simulink library "aerolibgravity2"  (R2020a)
settings: Solver=ode45  StartTime=0.0  StopTime=10.0  RelTol=1e-3
PostLoadFcn:
  | load_system('aerolibv1')
  | setsysloc('aerolibv1')
undefined symbols (not defined in the file or in its folder): aeroassertmsg, C, geoidgrid, ghCurrent, GM, latbp, lonbp, minYearCurrent, Newton, nMax10, nMax13, nMaxBetween, nMaxCurrent, R, Raphson, S, svCurrent, tabNMax10, tabNMax13, tabNMaxBetween
libraries: simulink x17, aerolibgravitysys x4
(part 1 of 4)
Description:
  | Aerospace Blockset Library: Gravity
settings Model: FPTRunName=Active  ExtModeAutoUpdateStatusClock=off  Creator=The MathWorks, Inc.  LastModifiedBy=The MathWorks, Inc.
settings DataIOCC: LimitDataPoints=on  SaveFormat=Array  SignalLoggingSaveFormat=ModelDataLogs  ReturnWorkspaceOutputs=off
settings OptimizationCC: BlockReduction=off  BooleanDataType=off  ExpressionDepthLimit=2147483647  EfficientMapNaN2IntZero=off  LifeSpan=inf
settings DebuggingCC: SaveWithParameterizedLinksMsg=none  UnderspecifiedInitializationDetection=Classic  MergeDetectMultiDrivingBlocksExec=none  SignalResolutionControl=TryResolveAllWithWarning  FcnCallInpInsideContextMsg=warning  AllowSymbolicDim=off  StateNameClashWarn=warning  SFUnexpectedBacktrackingDiag=warning  SFNoUnconditionalDefaultTransitionDiag=warning  SFExecutionAtInitializationDiag=none  ArithmeticOperatorsInVariantConditions=warning
settings HardwareCC: ProdBitPerPointer=32  ProdLargestAtomicFloat=None  ProdIntDivRoundTo=Undefined  ProdEndianess=Unspecified  ProdWordSize=32  ProdHWDeviceType=Specified  TargetUnknown=on
settings ModelReferenceCC: PropagateSignalLabelsOutOfModel=off
settings SFSimCC: SimUseLocalCustomCode=off  CustomCodeUndefinedFunction=UseInterfaceOnly
settings RTWCC: RTWUseLocalCustomCode=off
settings CodeAppCC: StateflowObjectComments=on
settings GRTTargetCC: TargetLangStandard=C89/C90 (ANSI)  CombineOutputUpdateFcns=off  GRTInterface=on
settings ConfigComp: CovMetricSettings=dw  CovHtmlReporting=on  CovSaveCumulativeToWorkspaceVar=on  CovSaveSingleToWorkspaceVar=on  CovExternalEMLEnable=off

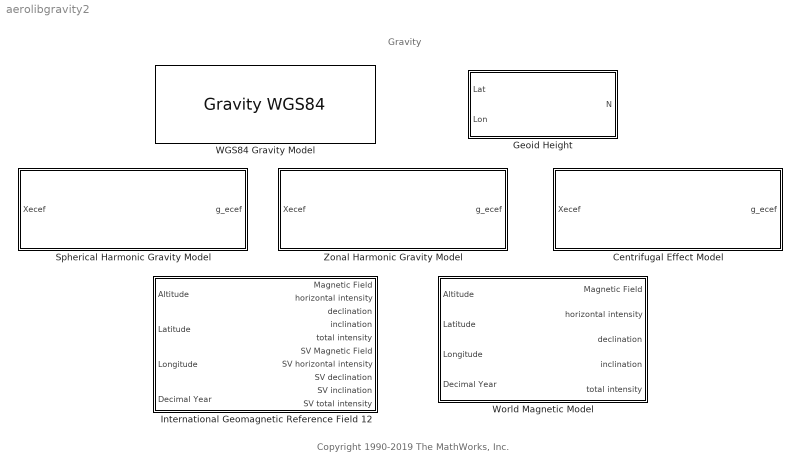
== system aerolibgravity2 ==
  note: Gravity
  note: Copyright 1990-2019 The MathWorks, Inc.
  Centrifugal Effect Model : Subsystem  BlockKeywords=__PRM__SERIALIZED__DATA__:centrifugal force,centrifugal acceleration,Mars,Moon,planet,Mercury,Venus,Jupiter,Saturn,Neptune,Uranus,gravity,rotation,Earth rotation,planetary rotation,non-inertial,noninertial,non inertial  mask(Centrifugal Effect Model){ptype=Earth, omega=7.2921150e-05, rate_loc=off}
      mask prompts: ptype "aeroblks:aeroblkgravity:blockCentrifugalEffectModelParamPlanetmodel"; omega "aeroblks:aeroblkgravity:blockCentrifugalEffectModelParamPlanetaryrotationalrateradsec"; rate_loc "aeroblks:aeroblkgravity:blockCentrifugalEffectModelParamInputplanetaryrotationalrate"
      mask help: aeroblks:aeroblkgravity:blockCentrifugalEffectModelDesc
      mask init:
      | [ports]=aeroicon('aeroblkcentrifugal','icon');
      mask Help: eval('asbhelp');
      mask TypeOptions ptype: aeroblks:aeroblkgravity:blockCentrifugalEffectModelParamComboMercury | aeroblks:aeroblkgravity:blockCentrifugalEffectModelParamComboVenus | aeroblks:aeroblkgravity:blockCentrifugalEffectModelParamComboEarth | aeroblks:aeroblkgravity:blockCentrifugalEffectModelParamComboMoon | aeroblks:aeroblkgravity:blockCentrifugalEffectModelParamComboMars | aeroblks:aeroblkgravity:blockCentrifugalEffectModelParamComboJupiter | aeroblks:aeroblkgravity:blockCentrifugalEffectModelParamComboSaturn | aeroblks:aeroblkgravity:blockCentrifugalEffectModelParamComboUranus | aeroblks:aeroblkgravity:blockCentrifugalEffectModelParamComboNeptune | aeroblks:aeroblkgravity:blockCentrifugalEffectModelParamComboCustom
      mask Callback ptype: aeroicon('aeroblkcentrifugal');
      mask Callback rate_loc: aeroicon('aeroblkcentrifugal');
      mask DialogControl ptype Prompt: Planet model:
      mask DialogControl omega Prompt: Planetary rotational rate [rad/sec]:
      mask DialogControl rate_loc Prompt: Input planetary rotational rate
      mask Display:
      | port_label(ports(1).type,ports(1).port,ports(1).txt,'texmode','on');
      | port_label(ports(2).type,ports(2).port,ports(2).txt,'texmode','on');
      | port_label(ports(3).type,ports(3).port,ports(3).txt,'texmode','on');
  Geoid Height : Subsystem  BlockKeywords=__PRM__SERIALIZED__DATA__:geoidheight,EGM96,EGM2008,geopotential model,WGS84 ellipsoid  mask(Geoid Height){units=Metric (MKS), gtype=EGM96, datafile='geoidegm96grid', dtype=double, action=Warning}
      mask prompts: units "aeroblks:aeroblkgravity:blockGeoidHeightParamUnits"; gtype "aeroblks:aeroblkgravity:blockGeoidHeightParamGeopotentialmodel"; datafile "aeroblks:aeroblkgravity:blockGeoidHeightParamGeopotentialmatfile"; dtype "aeroblks:aeroblkgravity:blockGeoidHeightParamDatatype"; action "aeroblks:aeroblkgravity:blockGeoidHeightParamActionforoutofrangeinput"
      mask help: aeroblks:aeroblkgravity:blockGeoidHeightDesc
      mask init:
      | [ports, latbp, lonbp, geoidgrid, errMode, errData, errSize] = aeroicon('aeroblkgeoidheight','icon');
      | blk = gcb;
      | switch errMode
      |     case 0
      |         % do nothing
      |     case 1
      |         error(message('aeroblks:aeroblkgeoidheight:noDataFile',...
      |                     datafile, blk));
      |     case 2
      |         error(message('aeroblks:aeroblkgeoidheight:noLatBP', ...
      |                     datafile, blk))
      |     case 3
      |         error(message('aeroblks:aeroblkgeoidheight:noLonBP', ...
      |                     datafile, blk))
      |     case 4
      |         error(message('aeroblks:aeroblkgeoidheight:noGrid', ...
      |                     datafile, blk))
      | end
      | switch errData
      |     case 0
      |         % do nothing
      |     case 1
      |         error(message('aeroblks:aeroblkgeoidheight:dataTypeLatLonGrid'));
      | end
      | switch errSize
      |     case 0
      |         % do nothing
      |     case 1
      |         error(message('aeroblks:aeroblkgeoidheight:sizeLatLon'));
      |     case 2
      |         error(message('aeroblks:aeroblkgeoidheight:sizeGrid'))
      |     case 3
      |         error(message('aeroblks:aeroblkgeoidheight:sizeLatLonGrid'))
      | end
      settings: AttributesFormatString=EGM2008 Geoid Data Unavailable
      mask Help: eval('asbhelp');
      mask TypeOptions units: aeroblks:aeroblkgravity:blockGeoidHeightParamComboMetricMKS | aeroblks:aeroblkgravity:blockGeoidHeightParamComboEnglish
      mask TypeOptions gtype: aeroblks:aeroblkgravity:blockGeoidHeightParamComboEGM96 | aeroblks:aeroblkgravity:blockGeoidHeightParamComboEGM2008 | aeroblks:aeroblkgravity:blockGeoidHeightParamComboCustom
      mask Callback gtype: aeroicon('aeroblkgeoidheight');
      mask TypeOptions dtype: aeroblks:aeroblkgravity:blockGeoidHeightParamCombodouble | aeroblks:aeroblkgravity:blockGeoidHeightParamCombosingle
      mask TypeOptions action: aeroblks:aeroblkgravity:blockGeoidHeightParamComboNone | aeroblks:aeroblkgravity:blockGeoidHeightParamComboWarning | aeroblks:aeroblkgravity:blockGeoidHeightParamComboError
      mask DialogControl units Prompt: Units:
      mask DialogControl gtype Prompt: Geopotential model:
      mask DialogControl getdata Prompt: aeroblks:aeroblkgeoidheight:getDataButton
      mask DialogControl getdata Callback: aeroDataPackage
      mask DialogControl datafile Prompt: Geopotential mat-file:
      mask DialogControl dtype Prompt: Data type:
      mask DialogControl action Prompt: Action for out-of-range input:
      mask Display:
      | port_label(ports(1).type,ports(1).port,ports(1).txt,'texmode','on');
      | port_label(ports(2).type,ports(2).port,ports(2).txt,'texmode','on');
      | port_label(ports(3).type,ports(3).port,ports(3).txt,'texmode','on');
  International Geomagnetic Reference Field 12 : Subsystem  BlockKeywords=__PRM__SERIALIZED__DATA__:IGRF,IGRF12,IGRF-12,IGRF 12,NOAA,magnetic field,secular variation,horizontal intensity,declination,inclination,sv,total intensity,tesla,nanotesla,Earth magnetic field  mask(InternationalGeomagneticReferenceField12){units=Metric (MKS), time_in=on, month=January, day=1, year=2020, action=None, sv_out=on}
      mask prompts: units "aeroblks:aeroblkgravity:blockInternationalGeomagneticReferenceField12ParamUnits"; time_in "aeroblks:aeroblkgravity:blockInternationalGeomagneticReferenceField12ParamInputdecimalyear"; month "aeroblks:aeroblkgravity:blockInternationalGeomagneticReferenceField12ParamMonth"; day "aeroblks:aeroblkgravity:blockInternationalGeomagneticReferenceField12ParamDay"; year "aeroblks:aeroblkgravity:blockInternationalGeomagneticReferenceField12ParamYear"; action "aeroblks:aeroblkgravity:blockInternationalGeomagneticReferenceField12ParamActionforoutofrangeinput"; sv_out "aeroblks:aeroblkgravity:blockInternationalGeomagneticReferenceField12ParamOutputsecularvariation"
      mask help: aeroblks:aeroblkgravity:blockInternationalGeomagneticReferenceField12Desc
      mask init:
      | [ports,dyear,tabNMax10,bpNMax10,nMax10,tabNMax13,bpNMax13,nMax13,...
      |    tabNMaxBetween,bpNMaxBetween,nMaxBetween,nMaxCurrent,minYearCurrent,...
      |    ghCurrent,svCurrent]=aeroicon('aeroblkigrf12','icon');
      | 
      | nPG = (nMax13*(nMax13+3))/2;
      mask Help: eval('asbhelp');
      mask TypeOptions units: aeroblks:aeroblkgravity:blockInternationalGeomagneticReferenceField12ParamComboMetricMKS | aeroblks:aeroblkgravity:blockInternationalGeomagneticReferenceField12ParamComboEnglish
      mask Callback time_in: aeroicon('aeroblkigrf12');
      mask TypeOptions month: aeroblks:aeroblkgravity:blockInternationalGeomagneticReferenceField12ParamComboJanuary | aeroblks:aeroblkgravity:blockInternationalGeomagneticReferenceField12ParamComboFebruary | aeroblks:aeroblkgravity:blockInternationalGeomagneticReferenceField12ParamComboMarch | aeroblks:aeroblkgravity:blockInternationalGeomagneticReferenceField12ParamComboApril | aeroblks:aeroblkgravity:blockInternationalGeomagneticReferenceField12ParamComboMay | aeroblks:aeroblkgravity:blockInternationalGeomagneticReferenceField12ParamComboJune | aeroblks:aeroblkgravity:blockInternationalGeomagneticReferenceField12ParamComboJuly | aeroblks:aeroblkgravity:blockInternationalGeomagneticReferenceField12ParamComboAugust | aeroblks:aeroblkgravity:blockInternationalGeomagneticReferenceField12ParamComboSeptember | aeroblks:aeroblkgravity:blockInternationalGeomagneticReferenceField12ParamComboOctober | aeroblks:aeroblkgravity:blockInternationalGeomagneticReferenceField12ParamComboNovember | aeroblks:aeroblkgravity:blockInternationalGeomagneticReferenceField12ParamComboDecember
      mask Callback month: aeroicon('aeroblkigrf12');
      mask TypeOptions day: 1 | 2 | 3 | 4 | 5 | 6 | 7 | 8 | 9 | 10 | 11 | 12 | 13 | 14 | 15 | 16 | 17 | 18 | 19 | 20 | 21 | 22 | 23 | 24 | 25 | 26 | 27 | 28 | 29 | 30 | 31
      mask Callback day: aeroicon('aeroblkigrf12');
      mask TypeOptions year: 2020 | 2019 | 2018 | 2017 | 2016 | 2015 | 2014 | 2013 | 2012 | 2011 | 2010 | 2009 | 2008 | 2007 | 2006 | 2005 | 2004 | 2003 | 2002 | 2001 | 2000 | 1999 | 1998 | 1997 | 1996 | 1995 | 1994 | 1993 | 1992 | 1991 | 1990 | 1989 | 1988 | 1987 | 1986 | 1985 | 1984 | 1983 | 1982 | 1981 | 1980 | 1979 | 1978 | 1977 | 1976 | 1975 | 1974 | 1973 | 1972 | 1971 | 1970 | 1969 | 1968 | 1967 | 1966 | 1965 | 1964 | 1963 | 1962 | 1961 | 1960 | 1959 | 1958 | 1957 | 1956 | 1955 | 1954 | 1953 | 1952 | 1951 | 1950 | 1949 | 1948 | 1947 | 1946 | 1945 | 1944 | 1943 | 1942 | 1941 | 1940 | 1939 | 1938 | 1937 | 1936 | 1935 | 1934 | 1933 | 1932 | 1931 | 1930 | 1929 | 1928 | 1927 | 1926 | 1925 | 1924 | 1923 | 1922 | 1921 | 1920 | 1919 | 1918 | 1917 | 1916 | 1915 | 1914 | 1913 | 1912 | 1911 | 1910 | 1909 | 1908 | 1907 | 1906 | 1905 | 1904 | 1903 | 1902 | 1901 | 1900
      mask Callback year: aeroicon('aeroblkigrf12');
      mask TypeOptions action: aeroblks:aeroblkgravity:blockInternationalGeomagneticReferenceField12ParamComboNone | aeroblks:aeroblkgravity:blockInternationalGeomagneticReferenceField12ParamComboWarning | aeroblks:aeroblkgravity:blockInternationalGeomagneticReferenceField12ParamComboError
      mask DialogControl units Prompt: Units:
      mask DialogControl time_in Prompt: Input decimal year
      mask DialogControl month Prompt: Month:
      mask DialogControl day Prompt: Day:
      mask DialogControl year Prompt: Year:
      mask DialogControl action Prompt: Action for out-of-range input:
      mask DialogControl sv_out Prompt: Output secular variation
      mask Display:
      | port_label(ports(1).type,ports(1).port,ports(1).txt);
      | port_label(ports(2).type,ports(2).port,ports(2).txt,'texmode','on');
      | port_label(ports(3).type,ports(3).port,ports(3).txt,'texmode','on');
      | port_label(ports(4).type,ports(4).port,ports(4).txt);
      | port_label(ports(5).type,ports(5).port,ports(5).txt);
      | port_label(ports(6).type,ports(6).port,ports(6).txt);
      | port_label(ports(7).type,ports(7).port,ports(7).txt);
      | port_label(ports(8).type,ports(8).port,ports(8).txt);
      | port_label(ports(9).type,ports(9).port,ports(9).txt);
      | port_label(ports(10).type,ports(10).port,ports(10).txt);
      | port_label(ports(11).type,ports(11).port,ports(11).txt);
      | port_label(ports(12).type,ports(12).port,ports(12).txt);
      | port_label(ports(13).type,ports(13).port,ports(13).txt);
      | port_label(ports(14).type,ports(14).port,ports(14).txt);
  Spherical Harmonic Gravity Model : Subsystem  BlockKeywords=__PRM__SERIALIZED__DATA__:planetary gravity,Earth gravity,EGM96,EGM2008,LP100K,LP165P,GMM2B,EIGENGL04C,harmonics,geopotential model,gravitational field,J2,J4,satellite,CubeSat,Mars gravity,Moon gravity,oblateness  mask(Spherical Harmonic Gravity Model){units=Metric (MKS), degree=120, action=Warning, ptype=EGM2008, datafile='aerogmm2b.mat'}
      mask prompts: units "aeroblks:aeroblkgravity:blockSphericalHarmonicGravityModelParamUnits"; degree "aeroblks:aeroblkgravity:blockSphericalHarmonicGravityModelParamDegree"; action "aeroblks:aeroblkgravity:blockSphericalHarmonicGravityModelParamActionforoutofrangeinput"; ptype "aeroblks:aeroblkgravity:blockSphericalHarmonicGravityModelParamPlanetmodel"; datafile "aeroblks:aeroblkgravity:blockSphericalHarmonicGravityModelParamPlanetmatfile"
      mask help: aeroblks:aeroblkgravity:blockSphericalHarmonicGravityModelDesc
      mask init:
      | [ports, maxdef, R, GM, Call, Sall, C, S]=aeroicon('aeroblkspherical','icon');
      mask Help: eval('asbhelp');
      mask TypeOptions units: aeroblks:aeroblkgravity:blockSphericalHarmonicGravityModelParamComboMetricMKS | aeroblks:aeroblkgravity:blockSphericalHarmonicGravityModelParamComboEnglish
      mask Callback degree: aeroicon('aeroblkspherical');
      mask TypeOptions action: aeroblks:aeroblkgravity:blockSphericalHarmonicGravityModelParamComboNone | aeroblks:aeroblkgravity:blockSphericalHarmonicGravityModelParamComboWarning | aeroblks:aeroblkgravity:blockSphericalHarmonicGravityModelParamComboError
      mask TypeOptions ptype: aeroblks:aeroblkgravity:blockSphericalHarmonicGravityModelParamComboEGM2008 | aeroblks:aeroblkgravity:blockSphericalHarmonicGravityModelParamComboEGM96 | aeroblks:aeroblkgravity:blockSphericalHarmonicGravityModelParamComboLP100K | aeroblks:aeroblkgravity:blockSphericalHarmonicGravityModelParamComboLP165P | aeroblks:aeroblkgravity:blockSphericalHarmonicGravityModelParamComboGMM2B | aeroblks:aeroblkgravity:blockSphericalHarmonicGravityModelParamComboCustom | aeroblks:aeroblkgravity:blockSphericalHarmonicGravityModelParamComboEIGENGL04C
      mask Callback ptype: aeroicon('aeroblkspherical');
      mask DialogControl ParameterTabVar0 Prompt: Main
      mask DialogControl units Prompt: Units:
      mask DialogControl degree Prompt: Degree:
      mask DialogControl action Prompt: Action for out-of-range input:
      mask DialogControl ParameterTabVar01 Prompt: Planet
      mask DialogControl ptype Prompt: Planet model:
      mask DialogControl datafile Prompt: Planet mat-file:
      mask Display:
      | port_label(ports(1).type,ports(1).port,ports(1).txt,'texmode','on');
      | port_label(ports(2).type,ports(2).port,ports(2).txt,'texmode','on');
  "WGS84 Gravity Model  " : GravityWGS84  BlockKeywords=__PRM__SERIALIZED__DATA__:world geodetic system,WGS 84,geocentric,equipotential,ellipsoid,WGS84 taylor series,WGS84 close approximation,WGS84 exact,Earth,1984,Earth gravity,planetary gravity,gravitational field
  World Magnetic Model : Subsystem  BlockKeywords=__PRM__SERIALIZED__DATA__:WMM,WMM2000,WMM-2000,WMM 2000,WMM2005,WMM-2005,WMM 2005,WMM2010,WMM-2010,WMM 2010,WMM2015,WMM-2015,WMM 2015,WMM2015v1,WMM-2015v1,WMM 2015v1,WMM 2015 v1,WMM2015v2,WMM-2015v2,WMM 2015v2,WMM 2015 v2,NOAA,magnetic field,horizontal intensity,declination,inclination,total intensity,tesla,nanotesla,Earth magnetic field  mask(WorldMagneticModel){model=WMM2020 (2020-2025), customFile='WMM2020.COF', units=Metric (MKS), time_in=on, month=January, day=1, year=2020, action=Error, h_out=on, dec_out=on, inc_out=on, ti_out=on}
      mask prompts: model "aeroblks:aeroblkgravity:blockWorldMagneticModelWMMCoeff"; customFile "aeroblks:aeroblkgravity:blockWorldMagneticModelCustomFile"; units "aeroblks:aeroblkgravity:blockWorldMagneticModel2015ParamUnits"; time_in "aeroblks:aeroblkgravity:blockWorldMagneticModel2015ParamInputdecimalyear"; month "aeroblks:aeroblkgravity:blockWorldMagneticModel2015ParamMonth"; day "aeroblks:aeroblkgravity:blockWorldMagneticModel2015ParamDay"; year "aeroblks:aeroblkgravity:blockWorldMagneticModel2015ParamYear"; action "aeroblks:aeroblkgravity:blockWorldMagneticModel2015ParamActionforoutofrangeinput"; h_out "aeroblks:aeroblkgravity:blockWorldMagneticModel2015ParamOutputhorizontalintensity"; dec_out "aeroblks:aeroblkgravity:blockWorldMagneticModel2015ParamOutputdeclination"; inc_out "aeroblks:aeroblkgravity:blockWorldMagneticModel2015ParamOutputinclination"; ti_out "aeroblks:aeroblkgravity:blockWorldMagneticModel2015ParamOutputtotalintensity"
      mask help: aeroblks:aeroblkgravity:blockWorldMagneticModel2020Desc
      mask init:
      | [ports,dyear,maxdef,epoch,c,cd,fn,fm,snorm,k]=aeroicon('aeroblkwmm','icon', model, year, month, day);
      settings: AttributesFormatString=%<model>
      mask Help: eval('asbhelp');
      mask TypeOptions model: aeroblks:aeroblkgravity:blockWorldMagneticModelWMMModel2000 | aeroblks:aeroblkgravity:blockWorldMagneticModelWMMModel2005 | aeroblks:aeroblkgravity:blockWorldMagneticModelWMMModel2010 | aeroblks:aeroblkgravity:blockWorldMagneticModelWMMModel2015v1 | aeroblks:aeroblkgravity:blockWorldMagneticModelWMMModel2015v2 | aeroblks:aeroblkgravity:blockWorldMagneticModelWMMModel2020 | aeroblks:aeroblkgravity:blockWorldMagneticModelWMMModelCustom
      mask Callback model: aeroicon('aeroblkwmm');
      mask TypeOptions units: aeroblks:aeroblkgravity:blockWorldMagneticModel2015ParamComboMetricMKS | aeroblks:aeroblkgravity:blockWorldMagneticModel2015ParamComboEnglish
      mask Callback time_in: aeroicon('aeroblkwmm');
      mask TypeOptions month: aeroblks:aeroblkgravity:blockWorldMagneticModel2015ParamComboJanuary | aeroblks:aeroblkgravity:blockWorldMagneticModel2015ParamComboFebruary | aeroblks:aeroblkgravity:blockWorldMagneticModel2015ParamComboMarch | aeroblks:aeroblkgravity:blockWorldMagneticModel2015ParamComboApril | aeroblks:aeroblkgravity:blockWorldMagneticModel2015ParamComboMay | aeroblks:aeroblkgravity:blockWorldMagneticModel2015ParamComboJune | aeroblks:aeroblkgravity:blockWorldMagneticModel2015ParamComboJuly | aeroblks:aeroblkgravity:blockWorldMagneticModel2015ParamComboAugust | aeroblks:aeroblkgravity:blockWorldMagneticModel2015ParamComboSeptember | aeroblks:aeroblkgravity:blockWorldMagneticModel2015ParamComboOctober | aeroblks:aeroblkgravity:blockWorldMagneticModel2015ParamComboNovember | aeroblks:aeroblkgravity:blockWorldMagneticModel2015ParamComboDecember
      mask Callback month: aeroicon('aeroblkwmm');
      mask TypeOptions day: 1 | 2 | 3 | 4 | 5 | 6 | 7 | 8 | 9 | 10 | 11 | 12 | 13 | 14 | 15 | 16 | 17 | 18 | 19 | 20 | 21 | 22 | 23 | 24 | 25 | 26 | 27 | 28 | 29 | 30 | 31
      mask Callback day: aeroicon('aeroblkwmm');
      mask Callback year: aeroicon('aeroblkwmm');
      mask TypeOptions action: aeroblks:aeroblkgravity:blockWorldMagneticModel2015ParamComboNone | aeroblks:aeroblkgravity:blockWorldMagneticModel2015ParamComboWarning | aeroblks:aeroblkgravity:blockWorldMagneticModel2015ParamComboError
      mask DialogControl Container3 Prompt: Model
      mask DialogControl model Prompt: WMM coefficients:
      mask DialogControl customFile Prompt: Custom .COF file:
      mask DialogControl units Prompt: Units:
      mask DialogControl time_in Prompt: Input decimal year
      mask DialogControl month Prompt: Month:
      mask DialogControl day Prompt: Day:
      mask DialogControl year Prompt: Year:
      mask DialogControl action Prompt: Action for out-of-range input:
      mask DialogControl h_out Prompt: Output horizontal intensity
      mask DialogControl dec_out Prompt: Output declination
      mask DialogControl inc_out Prompt: Output inclination
      mask DialogControl ti_out Prompt: Output total intensity
      mask Display:
      | port_label(ports(1).type,ports(1).port,ports(1).txt);
      | port_label(ports(2).type,ports(2).port,ports(2).txt,'texmode','on');
      | port_label(ports(3).type,ports(3).port,ports(3).txt,'texmode','on');
      | port_label(ports(4).type,ports(4).port,ports(4).txt);
      | port_label(ports(5).type,ports(5).port,ports(5).txt);
      | port_label(ports(6).type,ports(6).port,ports(6).txt);
      | port_label(ports(7).type,ports(7).port,ports(7).txt);
      | port_label(ports(8).type,ports(8).port,ports(8).txt);
      | port_label(ports(9).type,ports(9).port,ports(9).txt);
  Zonal Harmonic Gravity Model : Subsystem  BlockKeywords=__PRM__SERIALIZED__DATA__:planetary gravity,Earth gravity,harmonics,gravitational field,J2,J4,satellite,CubeSat,Mars gravity,Moon gravity,Mercury gravity,Venus gravity,Jupiter gravity,Saturn gravity,Neptune gravity,Uranus gravity,oblateness,J2,J3,J4  mask(Zonal Harmonic Gravity Model){units=Metric (MKS), degree=4, action=Warning, ptype=Earth, R=6378136.3, GM=398600441500000, jvalue=[1.0826269e-03 -2.5323000e-06 -1.6204000e-06]}
      mask prompts: units "aeroblks:aeroblkgravity:blockZonalHarmonicGravityModelParamUnits"; degree "aeroblks:aeroblkgravity:blockZonalHarmonicGravityModelParamDegree"; action "aeroblks:aeroblkgravity:blockZonalHarmonicGravityModelParamActionforoutofrangeinput"; ptype "aeroblks:aeroblkgravity:blockZonalHarmonicGravityModelParamPlanetmodel"; R "aeroblks:aeroblkgravity:blockZonalHarmonicGravityModelParamEquatorialradius"; GM "aeroblks:aeroblkgravity:blockZonalHarmonicGravityModelParamGravitationalparameter"; jvalue "aeroblks:aeroblkgravity:blockZonalHarmonicGravityModelParamJvalues"
      mask help: aeroblks:aeroblkgravity:blockZonalHarmonicGravityModelDesc
      mask init:
      | [ports]=aeroicon('aeroblkzonal','icon');
      mask Help: eval('asbhelp');
      mask TypeOptions units: aeroblks:aeroblkgravity:blockZonalHarmonicGravityModelParamComboMetricMKS | aeroblks:aeroblkgravity:blockZonalHarmonicGravityModelParamComboEnglish
      mask TypeOptions degree: aeroblks:aeroblkgravity:blockZonalHarmonicGravityModelParamCombo2 | aeroblks:aeroblkgravity:blockZonalHarmonicGravityModelParamCombo3 | aeroblks:aeroblkgravity:blockZonalHarmonicGravityModelParamCombo4
      mask Callback degree: aeroicon('aeroblkzonal');
      mask TypeOptions action: aeroblks:aeroblkgravity:blockZonalHarmonicGravityModelParamComboNone | aeroblks:aeroblkgravity:blockZonalHarmonicGravityModelParamComboWarning | aeroblks:aeroblkgravity:blockZonalHarmonicGravityModelParamComboError
      mask TypeOptions ptype: aeroblks:aeroblkgravity:blockZonalHarmonicGravityModelParamComboMercury | aeroblks:aeroblkgravity:blockZonalHarmonicGravityModelParamComboVenus | aeroblks:aeroblkgravity:blockZonalHarmonicGravityModelParamComboEarth | aeroblks:aeroblkgravity:blockZonalHarmonicGravityModelParamComboMoon | aeroblks:aeroblkgravity:blockZonalHarmonicGravityModelParamComboMars | aeroblks:aeroblkgravity:blockZonalHarmonicGravityModelParamComboJupiter | aeroblks:aeroblkgravity:blockZonalHarmonicGravityModelParamComboSaturn | aeroblks:aeroblkgravity:blockZonalHarmonicGravityModelParamComboUranus | aeroblks:aeroblkgravity:blockZonalHarmonicGravityModelParamComboNeptune | aeroblks:aeroblkgravity:blockZonalHarmonicGravityModelParamComboCustom
      mask Callback ptype: aeroicon('aeroblkzonal');
      mask Callback jvalue: aeroicon('aeroblkzonal');
      mask DialogControl ParameterTabVar0 Prompt: Main
      mask DialogControl units Prompt: Units:
      mask DialogControl degree Prompt: Degree:
      mask DialogControl action Prompt: Action for out-of-range input:
      mask DialogControl ParameterTabVar01 Prompt: Planet
      mask DialogControl ptype Prompt: Planet model:
      mask DialogControl R Prompt: Equatorial radius:
      mask DialogControl GM Prompt: Gravitational parameter:
      mask DialogControl jvalue Prompt: J values:
      mask Display:
      | port_label(ports(1).type,ports(1).port,ports(1).txt,'texmode','on');
      | port_label(ports(2).type,ports(2).port,ports(2).txt,'texmode','on');

== system aerolibgravity2/Centrifugal Effect Model ==
  Xecef : Inport
  Matrix Concatenate : Concatenate  NumInputs=3  Mode=Multidimensional array  ConcatenateDimension=2
  Omega : Constant  Value=omega  OutDataTypeStr=Inherit: Inherit via back propagation
  gx : Product  Inputs=3  RndMeth=Zero
  gy : Product  Inputs=3  RndMeth=Zero
  gz : Gain  Gain=0
  x : Selector  NumberOfDimensions=2  InputPortWidth=3  IndexOptions=Select all,Index vector (dialog)  Indices=1,1  OutputSizes=1,1
  y : Selector  NumberOfDimensions=2  InputPortWidth=3  IndexOptions=Select all,Index vector (dialog)  Indices=2,2  OutputSizes=1,1
  z : Selector  NumberOfDimensions=2  InputPortWidth=3  IndexOptions=Select all,Index vector (dialog)  Indices=2,3  OutputSizes=1,1
  g_ecef : Outport  VectorParamsAs1DForOutWhenUnconnected=off
  wires:
  gz/1 -> Matrix Concatenate/3
  z/1 -> gz/1
  y/1 -> gy/3
  x/1 -> gx/1
  Omega/1 -> gx/3, gx/2, gy/1, gy/2
  gy/1 -> Matrix Concatenate/2
  gx/1 -> Matrix Concatenate/1
  Matrix Concatenate/1 -> g_ecef/1
  Xecef/1 -> z/1, y/1, x/1

== system aerolibgravity2/Geoid Height ==
  Lat : Inport  OutDataTypeStr=double
  Lon : Inport  Port=2  OutDataTypeStr=double
  Check Latitude : simulink/Model Verification/Check  Static Range  Description=-90 <= u <= 90  max=90  max_included=on  min=-90  min_included=on  enabled=on  callback=aeroassertmsg('aeroblkgeoidheight','latitude','+/-90','warning');  stopWhenAssertionFail=off  export=off  icon=graphic
      settings: SourceProductBaseCode=SL
  Check Longitude : simulink/Model Verification/Check  Static Range  Description=0 <= u <= 360  max=360  max_included=on  min=0  min_included=on  enabled=on  callback=aeroassertmsg('aeroblkgeoidheight','longitiude','0 to 360','warning');  stopWhenAssertionFail=off  export=off  icon=graphic
      settings: SourceProductBaseCode=SL
  Data Type Conversion : DataTypeConversion  OutDataTypeStr=single
  Data Type Conversion1 : DataTypeConversion  OutDataTypeStr=single
  Disallow CGS : UnitConfiguration  UnitSystemsStr=English,SI,SI (extended)  AllowAllUnitSystems=off
  Format Output : Subsystem
  Lookup Table (n-D) : Lookup_n-D  BreakpointsForDimension1=latbp  BreakpointsForDimension2=lonbp  IndexSearchMethod=Evenly spaced points  BeginIndexSearchUsingPreviousIndexResult=on  Table=geoidgrid  InterpMethod=Cubic spline  ExtrapMethod=Clip  InputSameDT=on
  Wrap Latitude : Subsystem
  Wrap Longitude : Subsystem
  N : Outport  OutDataTypeStr=double  Unit=m  VectorParamsAs1DForOutWhenUnconnected=off
  wires:
  Lookup Table (n-D)/1 -> Format Output/1(Lon)
  Format Output/1(Lon1) -> N/1
  Lat/1 -> Wrap Latitude/1(Lat), Check Latitude/1
  Lon/1 -> Wrap Latitude/2(Lon), Check Longitude/1
  Wrap Longitude/1(Lon1) -> Data Type Conversion/1
  Wrap Latitude/2(Lon1) -> Wrap Longitude/1(Lon)
  Wrap Latitude/1(Lat1) -> Data Type Conversion1/1
  Data Type Conversion1/1 -> Lookup Table (n-D)/1
  Data Type Conversion/1 -> Lookup Table (n-D)/2

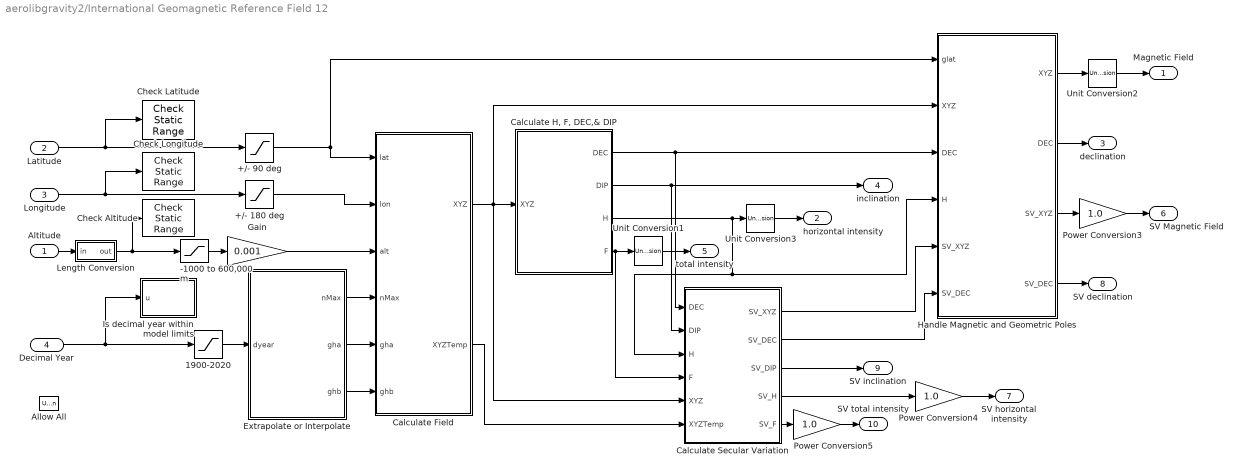
== system aerolibgravity2/International Geomagnetic Reference Field 12 ==
  Altitude : Inport  Unit=m
  Latitude : Inport  Port=2  Unit=deg
  Longitude : Inport  Port=3  Unit=deg
  Decimal Year : Inport  Port=4
  +/- 180 deg : Saturate  UpperLimit=180.0  LowerLimit=-180.0  OutDataTypeStr=Inherit: Inherit via back propagation
  +/- 90 deg : Saturate  UpperLimit=90.0  LowerLimit=-90.0  OutDataTypeStr=Inherit: Inherit via back propagation
  -1000 to 600,000 m : Saturate  UpperLimit=600000.0  LowerLimit=-1000  OutDataTypeStr=Inherit: Inherit via back propagation
  1900-2020 : Saturate  UpperLimit=2020  LowerLimit=1900  OutDataTypeStr=Inherit: Inherit via back propagation
  Allow All : UnitConfiguration  UnitSystemsStr=all  AllowAllUnitSystems=on
  Calculate Field : Subsystem
  "Calculate H, F, DEC,& DIP" : Subsystem
  Calculate Secular Variation : Subsystem
  Check Altitude : simulink/Model Verification/Check  Static Range  Description=-1000 <= u <= 600000  max=600000  max_included=on  min=-1000  min_included=on  enabled=off  callback=aeroassertmsg('aeroblkigrf','alt','none')  stopWhenAssertionFail=off  export=off  icon=graphic
      settings: SourceProductBaseCode=SL
  Check Latitude : simulink/Model Verification/Check  Static Range  Description=-90 <= u <= 90  max=90  max_included=on  min=-90  min_included=on  enabled=off  callback=aeroassertmsg('aeroblkigrf','lat','none')  stopWhenAssertionFail=off  export=off  icon=graphic
      settings: SourceProductBaseCode=SL
  Check Longitude : simulink/Model Verification/Check  Static Range  Description=-180 <= u <= 180  max=180  max_included=on  min=-180  min_included=on  enabled=off  callback=aeroassertmsg('aeroblkigrf','lon','none')  stopWhenAssertionFail=off  export=off  icon=graphic
      settings: SourceProductBaseCode=SL
  Extrapolate or Interpolate : Subsystem
  Gain : Gain  Gain=0.001  OutDataTypeStr=Inherit: Inherit via back propagation  SaturateOnIntegerOverflow=on
  Handle Magnetic and Geometric Poles : Subsystem
  Is decimal year within model limits : Subsystem  Description=1900 <= u <= 2020  mask(Checks_SRange){max=2020, max_included=on, min=1900, min_included=on, enabled=off, callback=aeroassertmsg('aeroblkigrf','time','none'), stopWhenAssertionFail=off, export=off, icon=graphic}
      mask prompts: max "Upper bound:"; max_included "Inclusive upper bound"; min "Lower bound:"; min_included "Inclusive lower bound"; enabled "Enable assertion"; callback "Simulation callback when assertion fails (optional):"; stopWhenAssertionFail "Stop simulation when assertion fails"; export "Output assertion signal"; icon "Select icon type:"
      mask help: Assert that the input signal lies between a static lower and upper bound or optionally equals either bound.
      mask init:
      | update_assert_sys(gcbh);
      mask TypeOptions icon: graphic | text
      mask Display:
      | plot([0 1], [0 1]);
      | plot([0 1],[1 0]);
  Length Conversion : Subsystem
  Power Conversion3 : Gain  Gain=1.0  OutDataTypeStr=Inherit: Inherit via back propagation  SaturateOnIntegerOverflow=on
  Power Conversion4 : Gain  Gain=1.0  OutDataTypeStr=Inherit: Inherit via back propagation  SaturateOnIntegerOverflow=on
  Power Conversion5 : Gain  Gain=1.0  OutDataTypeStr=Inherit: Inherit via back propagation  SaturateOnIntegerOverflow=on
  Unit Conversion1 : UnitConversion
  Unit Conversion2 : UnitConversion
  Unit Conversion3 : UnitConversion
  Magnetic Field : Outport  Unit=nT  VectorParamsAs1DForOutWhenUnconnected=off
  horizontal intensity : Outport  Port=2  Unit=nT  VectorParamsAs1DForOutWhenUnconnected=off
  declination : Outport  Port=3  Unit=deg  VectorParamsAs1DForOutWhenUnconnected=off
  inclination : Outport  Port=4  Unit=deg  VectorParamsAs1DForOutWhenUnconnected=off
  total intensity : Outport  Port=5  Unit=nT  VectorParamsAs1DForOutWhenUnconnected=off
  SV Magnetic Field : Outport  Port=6  VectorParamsAs1DForOutWhenUnconnected=off
  SV horizontal intensity : Outport  Port=7  VectorParamsAs1DForOutWhenUnconnected=off
  SV declination : Outport  Port=8  VectorParamsAs1DForOutWhenUnconnected=off
  SV inclination : Outport  Port=9  VectorParamsAs1DForOutWhenUnconnected=off
  SV total intensity : Outport  Port=10  VectorParamsAs1DForOutWhenUnconnected=off
  wires:
  Extrapolate or Interpolate/3(ghb) -> Calculate Field/6(ghb)
  Extrapolate or Interpolate/2(gha) -> Calculate Field/5(gha)
  Extrapolate or Interpolate/1(nMax) -> Calculate Field/4(nMax)
  Calculate Field/2(XYZTemp) -> Calculate Secular Variation/6(XYZTemp)
  "Calculate H, F, DEC,& DIP"/2(DIP) -> inclination/1, Calculate Secular Variation/2(DIP)
  "Calculate H, F, DEC,& DIP"/1(DEC) -> Handle Magnetic and Geometric Poles/3("DEC "), Calculate Secular Variation/1(DEC)
  Calculate Field/1(XYZ) -> Handle Magnetic and Geometric Poles/2("XYZ "), "Calculate H, F, DEC,& DIP"/1(XYZ), Calculate Secular Variation/5(XYZ)
  Power Conversion5/1 -> SV total intensity/1
  Power Conversion4/1 -> SV horizontal intensity/1
  Power Conversion3/1 -> SV Magnetic Field/1
  Altitude/1 -> Length Conversion/1(in)
  Length Conversion/1(out) -> -1000 to 600,000 m/1, Check Altitude/1
  Decimal Year/1 -> Is decimal year within model limits/1(u), 1900-2020/1
  Latitude/1 -> +/- 90 deg/1, Check Latitude/1
  Longitude/1 -> +/- 180 deg/1, Check Longitude/1
  Gain/1 -> Calculate Field/3(alt)
  Handle Magnetic and Geometric Poles/1(XYZ) -> Unit Conversion2/1
  "Calculate H, F, DEC,& DIP"/4(F) -> Unit Conversion1/1, Calculate Secular Variation/4(F)
  +/- 90 deg/1 -> Calculate Field/1(lat), Handle Magnetic and Geometric Poles/1(glat)
  +/- 180 deg/1 -> Calculate Field/2(lon)
  -1000 to 600,000 m/1 -> Gain/1
  Calculate Secular Variation/1(SV_XYZ) -> Handle Magnetic and Geometric Poles/5("SV_XYZ ")
  Calculate Secular Variation/4(SV_H) -> Power Conversion4/1
  Calculate Secular Variation/2(SV_DEC) -> Handle Magnetic and Geometric Poles/6("SV_DEC ")
  Calculate Secular Variation/3(SV_DIP) -> SV inclination/1
  Calculate Secular Variation/5(SV_F) -> Power Conversion5/1
  1900-2020/1 -> Extrapolate or Interpolate/1(dyear)
  Handle Magnetic and Geometric Poles/4(SV_DEC) -> SV declination/1
  Handle Magnetic and Geometric Poles/3(SV_XYZ) -> Power Conversion3/1
  Handle Magnetic and Geometric Poles/2(DEC) -> declination/1
  "Calculate H, F, DEC,& DIP"/3(H) -> Unit Conversion3/1, Calculate Secular Variation/3(H), Handle Magnetic and Geometric Poles/4(H)
  Unit Conversion1/1 -> total intensity/1
  Unit Conversion2/1 -> Magnetic Field/1
  Unit Conversion3/1 -> horizontal intensity/1

== system aerolibgravity2/Spherical Harmonic Gravity Model ==
  Xecef : Inport  Unit=m
  Calculate gravity in ECEF frame : Subsystem
  Compute gravity in spherical coordinates : Subsystem
  Disallow CGS : UnitConfiguration  UnitSystemsStr=English,SI,SI (extended)  AllowAllUnitSystems=off
  "Find radius, geocentric latitude, and longitude" : Subsystem
  Get Cosine and Sine of Latitude and Longitude : Subsystem
  Is r above equatorial radius? : simulink/Model Verification/Check Static  Lower Bound  Description=R <= u  min=R  min_included=on  enabled=on  callback=aeroassertmsg('aeroblkspherical','warning');  stopWhenAssertionFail=off  export=off  icon=graphic
  sin(m_lon) & cos(m_lon) : Subsystem
  g_ecef : Outport  Unit=m/s^2  VectorParamsAs1DForOutWhenUnconnected=off
  wires:
  Get Cosine and Sine of Latitude and Longitude/3(trlat) -> Compute gravity in spherical coordinates/3(trlat)
  Calculate gravity in ECEF frame/1(g_ecef) -> g_ecef/1
  Compute gravity in spherical coordinates/1(dUdr dUdphi dUdlambda) -> Calculate gravity in ECEF frame/1(dUdr dUdphi dUdlambda)
  sin(m_lon) & cos(m_lon)/2(crlon_array) -> Compute gravity in spherical coordinates/2(crlon_array)
  Get Cosine and Sine of Latitude and Longitude/4(srphi) -> Compute gravity in spherical coordinates/4(srphi)
  Get Cosine and Sine of Latitude and Longitude/5(crphi) -> Compute gravity in spherical coordinates/5(crphi)
  sin(m_lon) & cos(m_lon)/1(srlon_array) -> Compute gravity in spherical coordinates/1(srlon_array)
  "Find radius, geocentric latitude, and longitude"/1(rlon) -> Get Cosine and Sine of Latitude and Longitude/1(rlon)
  Get Cosine and Sine of Latitude and Longitude/2(crlon) -> sin(m_lon) & cos(m_lon)/2(crlon)
  Get Cosine and Sine of Latitude and Longitude/1(srlon) -> sin(m_lon) & cos(m_lon)/1(srlon)
  "Find radius, geocentric latitude, and longitude"/3(r) -> Is r above equatorial radius?/1, Calculate gravity in ECEF frame/3(r), Compute gravity in spherical coordinates/6(r)
  "Find radius, geocentric latitude, and longitude"/2(rlat) -> Get Cosine and Sine of Latitude and Longitude/2(rlat), Calculate gravity in ECEF frame/2(rlat)
  Xecef/1 -> Calculate gravity in ECEF frame/4(Xecef), "Find radius, geocentric latitude, and longitude"/1(Xecef)

== system aerolibgravity2/World Magnetic Model ==
  Altitude : Inport  Unit=m
  Latitude : Inport  Port=2  Unit=deg
  Longitude : Inport  Port=3  Unit=deg
  Decimal Year : Inport  Port=4
  +/- 180 deg : Saturate  UpperLimit=180.0  LowerLimit=-180.0
  +/- 90 deg : Saturate  UpperLimit=90.0  LowerLimit=-90.0
  0 to 1,000,000 m : Saturate  UpperLimit=1000000.0  LowerLimit=0
  Allow All : UnitConfiguration  UnitSystemsStr=all  AllowAllUnitSystems=on
  Check Altitude : simulink/Model Verification/Check  Static Range  Description=0 <= u <= 1000000  max=1000000  max_included=on  min=0  min_included=on  enabled=on  callback=aeroassertmsg('aeroblkwmm','alt','error')  stopWhenAssertionFail=on  export=off  icon=graphic
      settings: SourceProductBaseCode=SL
  Check Latitude : simulink/Model Verification/Check  Static Range  Description=-90 <= u <= 90  max=90  max_included=on  min=-90  min_included=on  enabled=on  callback=aeroassertmsg('aeroblkwmm','lat','error')  stopWhenAssertionFail=on  export=off  icon=graphic
      settings: SourceProductBaseCode=SL
  Check Longitude : simulink/Model Verification/Check  Static Range  Description=-180 <= u <= 180  max=180  max_included=on  min=-180  min_included=on  enabled=on  callback=aeroassertmsg('aeroblkwmm','lon','error')  stopWhenAssertionFail=on  export=off  icon=graphic
      settings: SourceProductBaseCode=SL
  "Compute x,y,z, and h components of magnetic field" : aerolibgravitysys/Compute x,y,z, and h components of magnetic field  SystemSampleTime=-1  Latency=0  AutoFrameSizeCalculation=off
      settings: SourceProductBaseCode=AE
  Gain : Gain  Gain=0.001  SaturateOnIntegerOverflow=on  OutDataTypeStr=Inherit: Same as input  ParamDataTypeStr=Inherit: Same as input
  Is time within model limits : Subsystem  Description=0 <= u <= 5  mask(Checks_SRange){max=5, max_included=on, min=0, min_included=on, enabled=on, callback=aeroassertmsg('aeroblkwmm','time','error'), stopWhenAssertionFail=on, export=off, icon=graphic}
      mask prompts: max "Upper bound:"; max_included "Inclusive upper bound"; min "Lower bound:"; min_included "Inclusive lower bound"; enabled "Enable assertion"; callback "Simulation callback when assertion fails (optional):"; stopWhenAssertionFail "Stop simulation when assertion fails"; export "Output assertion signal"; icon "Select icon type:"
      mask help: Assert that the input signal lies between a static lower and upper bound or optionally equals either bound.
      mask init:
      | update_assert_sys(gcbh);
      mask TypeOptions icon: graphic | text
  Length Conversion : Subsystem
  MagField Conversion : Subsystem
  MagField Conversion1 : Subsystem
  Mux : Mux  Inputs=3
  Unit Conversion2 : UnitConversion
  geomag : aerolibgravitysys/geomag  SystemSampleTime=-1  Latency=0  AutoFrameSizeCalculation=off
      settings: SourceProductBaseCode=AE
  Magnetic Field : Outport  Unit=nT  VectorParamsAs1DForOutWhenUnconnected=off
  horizontal intensity : Outport  Port=2  Unit=nT  VectorParamsAs1DForOutWhenUnconnected=off
  declination : Outport  Port=3  Unit=deg  VectorParamsAs1DForOutWhenUnconnected=off
  inclination : Outport  Port=4  Unit=deg  VectorParamsAs1DForOutWhenUnconnected=off
  total intensity : Outport  Port=5  Unit=nT  VectorParamsAs1DForOutWhenUnconnected=off
  wires:
  Altitude/1 -> Length Conversion/1(in)
  Length Conversion/1(out) -> 0 to 1,000,000 m/1, Check Altitude/1
  "Compute x,y,z, and h components of magnetic field"/1 -> Mux/1
  "Compute x,y,z, and h components of magnetic field"/2 -> Mux/2
  "Compute x,y,z, and h components of magnetic field"/3 -> Mux/3
  "Compute x,y,z, and h components of magnetic field"/4 -> MagField Conversion/1(in)
  Decimal Year/1 -> geomag/1
  geomag/2 -> "Compute x,y,z, and h components of magnetic field"/2, inclination/1
  Latitude/1 -> +/- 90 deg/1, Check Latitude/1
  Longitude/1 -> +/- 180 deg/1, Check Longitude/1
  Gain/1 -> geomag/4
  geomag/1 -> "Compute x,y,z, and h components of magnetic field"/1, declination/1
  Mux/1 -> Unit Conversion2/1
  Unit Conversion2/1 -> Magnetic Field/1
  geomag/3 -> MagField Conversion1/1(in), "Compute x,y,z, and h components of magnetic field"/3
  MagField Conversion/1(out) -> horizontal intensity/1
  +/- 90 deg/1 -> geomag/3
  +/- 180 deg/1 -> geomag/2
  0 to 1,000,000 m/1 -> Gain/1
  geomag/4 -> Is time within model limits/1(u)
  MagField Conversion1/1(out) -> total intensity/1

== system aerolibgravity2/Zonal Harmonic Gravity Model ==
  Xecef : Inport  Unit=m
  Calculate Legendre functions : aerolibgravitysys/Calculate  Legendre functions Degree 4  SystemSampleTime=-1  Latency=0  AutoFrameSizeCalculation=off
      settings: SourceProductBaseCode=AE
  Calculate gravity in ECEF frame : Subsystem
  Calculate radial and transverse gravity : aerolibgravitysys/Calculate radial and transverse gravity Degree 4  SystemSampleTime=-1  Latency=0  AutoFrameSizeCalculation=off
      settings: SourceProductBaseCode=AE
  Disallow CGS : UnitConfiguration  UnitSystemsStr=English,SI,SI (extended)  AllowAllUnitSystems=off
  Find radius and geocentric latitude : Subsystem
  g_ecef : Outport  Unit=m/s^2  VectorParamsAs1DForOutWhenUnconnected=off
  wires:
  Calculate gravity in ECEF frame/1(g_ecef) -> g_ecef/1
  Calculate radial and transverse gravity/2 -> Calculate gravity in ECEF frame/2(g_trans)
  Calculate radial and transverse gravity/1 -> Calculate gravity in ECEF frame/1(g_radial)
  Calculate Legendre functions/1 -> Calculate radial and transverse gravity/1
  Find radius and geocentric latitude/2(r) -> Calculate radial and transverse gravity/2, Calculate gravity in ECEF frame/3(r)
  Find radius and geocentric latitude/1(rlat) -> Calculate Legendre functions/1
  Xecef/1 -> Calculate gravity in ECEF frame/4(Xecef), Find radius and geocentric latitude/1(Xecef)

== system aerolibgravity2/Geoid Height/Format Output ==
  Lon : Inport
  Change Units : Subsystem
  Data Type Conversion : DataTypeConversion  OutDataTypeStr=double
  Data Type Conversion1 : DataTypeConversion  OutDataTypeStr=double
  Truncate : Subsystem
  Truncate1 : Subsystem
  Lon1 : Outport  VectorParamsAs1DForOutWhenUnconnected=off
  wires:
  Truncate1/1(Out1) -> Change Units/1(in)
  Truncate/1(Out1) -> Data Type Conversion/1
  Change Units/1(out) -> Truncate/1(In1)
  Data Type Conversion1/1 -> Truncate1/1(In1)
  Data Type Conversion/1 -> Lon1/1
  Lon/1 -> Data Type Conversion1/1

== system aerolibgravity2/Geoid Height/Wrap Latitude ==
  Lat : Inport
  Lon : Inport  Port=2
  If : If  IfExpression=u1 == 0
  If Action Subsystem : Subsystem  TreatAsAtomicUnit=on
  If Action Subsystem1 : Subsystem  TreatAsAtomicUnit=on
  Interval Test : simulink/Logic and Bit Operations/Interval Test  IntervalClosedRight=on  uplimit=90  IntervalClosedLeft=on  lowlimit=-90  OutDataTypeStr=boolean
  Merge : Merge
  Merge1 : Merge
  Wrap Latitude 180 : Subsystem
  Lat1 : Outport  VectorParamsAs1DForOutWhenUnconnected=off
  Lon1 : Outport  Port=2  VectorParamsAs1DForOutWhenUnconnected=off
  wires:
  [latw0] -> Merge/1
  [latw1] -> Merge/2
  [lonw0] -> Merge1/1
  [lonw1] -> Merge1/2
  Lon/1 -> [lon]
  If/1 -> If Action Subsystem/Action
  Interval Test/1 -> If/1
  [lat] -> If Action Subsystem/1(Lat)
  [lon] -> If Action Subsystem/2(Lon)
  If/2 -> If Action Subsystem1/Action
  [lat] -> If Action Subsystem1/1(Lat)
  [lon] -> If Action Subsystem1/2(Lon)
  If Action Subsystem/1(Lat1) -> [latw0]
  If Action Subsystem1/1(Lat1) -> [latw1]
  If Action Subsystem1/2(Lon1) -> [lonw1]
  If Action Subsystem/2(Lon1) -> [lonw0]
  Merge/1 -> Lat1/1
  Merge1/1 -> Lon1/1
  Lat/1 -> Wrap Latitude 180/1(lat)
  Wrap Latitude 180/1(lat 180) -> Interval Test/1, [lat]

== system aerolibgravity2/Geoid Height/Wrap Longitude ==
  Lon : Inport
  If : If  IfExpression=u1 == 0
  If Action Subsystem : Subsystem  TreatAsAtomicUnit=on
  If Action Subsystem1 : Subsystem  TreatAsAtomicUnit=on
  Interval Test : simulink/Logic and Bit Operations/Interval Test  IntervalClosedRight=on  uplimit=360  IntervalClosedLeft=on  lowlimit=0  OutDataTypeStr=boolean
  Merge : Merge
  Lon1 : Outport  VectorParamsAs1DForOutWhenUnconnected=off
  wires:
  Lon/1 -> Interval Test/1, [lon]
  Interval Test/1 -> If/1
  If/1 -> If Action Subsystem/Action
  [lon] -> If Action Subsystem/1(Lon)
  Merge/1 -> Lon1/1
  If Action Subsystem/1(Lon1) -> Merge/1
  [lon] -> If Action Subsystem1/1(Lon)
  If/2 -> If Action Subsystem1/Action
  If Action Subsystem1/1(Lon1) -> Merge/2

== system aerolibgravity2/International Geomagnetic Reference Field 12/Calculate Field ==
  lat : Inport
  lon : Inport  Port=2
  alt : Inport  Port=3
  nMax : Inport  Port=4
  gha : Inport  Port=5
  ghb : Inport  Port=6
  Compute magnetic vector in spherical coordinates : Subsystem
  Convert from geodetic to spherical coordinates : Subsystem  TreatAsAtomicUnit=on
  Get Cosine and Sine of Latitude and Longitude : Subsystem
  Has altitude or latitude changed : Subsystem
  "Has longitude changed " : Subsystem
  Logical Operator : Logic  Operator=OR  AllPortsSameDT=off  OutDataTypeStr=boolean
  lat1 : InportShadow
  lon1 : InportShadow  Port=2
  XYZ : Outport  VectorParamsAs1DForOutWhenUnconnected=off
  XYZTemp : Outport  Port=2  VectorParamsAs1DForOutWhenUnconnected=off
  wires:
  Logical Operator/1 -> Get Cosine and Sine of Latitude and Longitude/Enable, Compute magnetic vector in spherical coordinates/Enable
  "Has longitude changed "/1(Longitude change) -> Logical Operator/1
  nMax/1 -> Compute magnetic vector in spherical coordinates/10(nMax)
  Get Cosine and Sine of Latitude and Longitude/1(srlat) -> Convert from geodetic to spherical coordinates/2(srlat)
  Get Cosine and Sine of Latitude and Longitude/2(srlat2) -> Convert from geodetic to spherical coordinates/3(srlat2)
  Get Cosine and Sine of Latitude and Longitude/3(crlat2) -> Convert from geodetic to spherical coordinates/4(crlat2)
  Get Cosine and Sine of Latitude and Longitude/4(crlat) -> Convert from geodetic to spherical coordinates/5(crlat)
  Has altitude or latitude changed/1(Alt_Lat change) -> Logical Operator/2, Convert from geodetic to spherical coordinates/Enable
  alt/1 -> Convert from geodetic to spherical coordinates/1(alt), Has altitude or latitude changed/2(alt)
  Convert from geodetic to spherical coordinates/1(r) -> Compute magnetic vector in spherical coordinates/3(r)
  lat/1 -> Has altitude or latitude changed/1(lat)
  lon/1 -> "Has longitude changed "/1(lon)
  lon1/1 -> Get Cosine and Sine of Latitude and Longitude/1(lon)
  lat1/1 -> Get Cosine and Sine of Latitude and Longitude/2(lat)
  Convert from geodetic to spherical coordinates/2(clat) -> Compute magnetic vector in spherical coordinates/4(clat)
  Convert from geodetic to spherical coordinates/3(slat) -> Compute magnetic vector in spherical coordinates/5(slat)
  Get Cosine and Sine of Latitude and Longitude/5(crlon) -> Compute magnetic vector in spherical coordinates/8(crlon)
  Get Cosine and Sine of Latitude and Longitude/6(srlon) -> Compute magnetic vector in spherical coordinates/9(srlon)
  Convert from geodetic to spherical coordinates/4(sd) -> Compute magnetic vector in spherical coordinates/6(sd)
  Convert from geodetic to spherical coordinates/5(cd) -> Compute magnetic vector in spherical coordinates/7(cd)
  gha/1 -> Compute magnetic vector in spherical coordinates/1(gha)
  ghb/1 -> Compute magnetic vector in spherical coordinates/2(ghb)
  Compute magnetic vector in spherical coordinates/1(XYZ) -> XYZ/1
  Compute magnetic vector in spherical coordinates/2(XYZTemp) -> XYZTemp/1

== system aerolibgravity2/International Geomagnetic Reference Field 12/Calculate H, F, DEC,& DIP ==
  XYZ : Inport
  "DEC " : Merge
  "DIP " : Merge
  Demux : Demux  Outputs=3
  Else Action : Subsystem  TreatAsAtomicUnit=on
  "F " : Sqrt  SaturateOnIntegerOverflow=on
  "H " : Sqrt  SaturateOnIntegerOverflow=on
  If : If  IfExpression=u1 < 0.0001
  If Action : Subsystem  TreatAsAtomicUnit=on
  Sum : Sum  Inputs=|++
  Sum1 : Sum  Inputs=|++
  X2 : Product  RndMeth=Zero
  Y2 : Product  RndMeth=Zero
  Z2 : Product  RndMeth=Zero
  DEC : Outport  Unit=deg  VectorParamsAs1DForOutWhenUnconnected=off
  DIP : Outport  Port=2  Unit=deg  VectorParamsAs1DForOutWhenUnconnected=off
  H : Outport  Port=3  Unit=nT  VectorParamsAs1DForOutWhenUnconnected=off
  F : Outport  Port=4  Unit=nT  VectorParamsAs1DForOutWhenUnconnected=off
  wires:
  X2/1 -> Sum/1
  Y2/1 -> Sum/2
  Sum/1 -> "H "/1, Sum1/1
  Z2/1 -> Sum1/2
  Sum1/1 -> "F "/1
  Demux/3 -> Z2/1, Z2/2, Else Action/1(Z)
  Demux/2 -> Y2/2, Y2/1, Else Action/2(Y)
  Demux/1 -> X2/2, X2/1, Else Action/3(X)
  "H "/1 -> H/1, Else Action/4(H)
  "F "/1 -> F/1, If/1
  If/1 -> If Action/Action
  If/2 -> Else Action/Action
  If Action/1(DEC) -> "DEC "/1
  Else Action/1(DEC) -> "DEC "/2
  "DEC "/1 -> DEC/1
  "DIP "/1 -> DIP/1
  If Action/2(DIP) -> "DIP "/1
  Else Action/2(DIP) -> "DIP "/2
  XYZ/1 -> Demux/1
